simulink model "ModeloSimulink"  (R2023a)
settings: Solver=VariableStepAuto  StartTime=0.0  StopTime=10000  MaxStep=0.1  RelTol=1e-3
settings Model: Creator=User  LastModifiedBy=dougl
settings DebuggingCC: UnconnectedInputMsg=warning  UnconnectedOutputMsg=warning  UnconnectedLineMsg=warning
settings ModelReferenceCC: EnableRefExpFcnMdlSchedulingChecks=on
settings RTWCC: DLArmComputeVersion=19.05

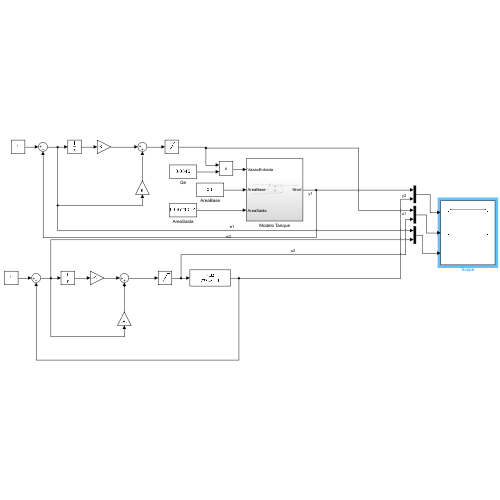
[thumbnail: Simulink's stored preview of the top-level diagram]
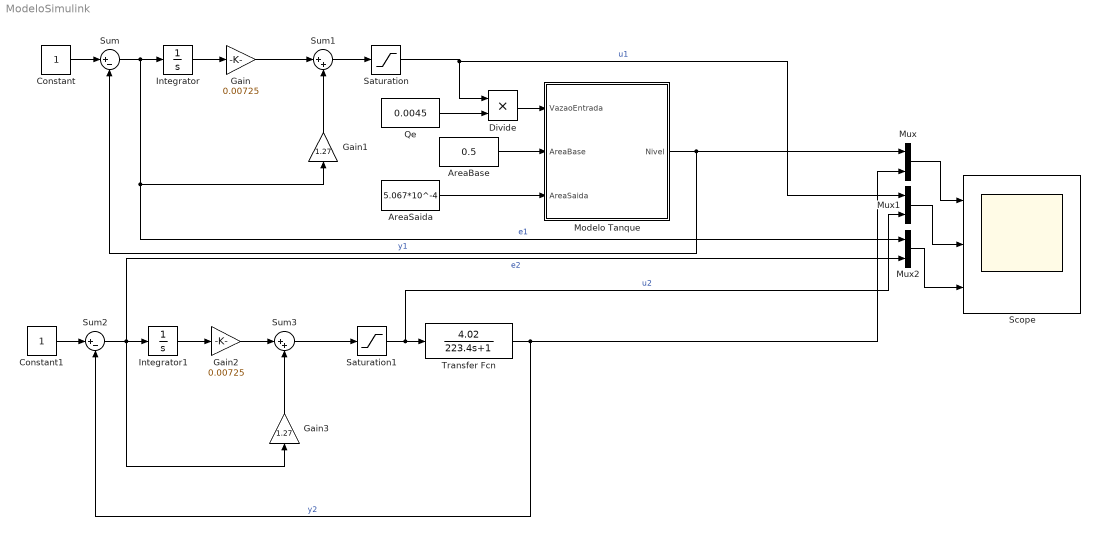
== system ModeloSimulink ==
  AreaBase : Constant  Value=0.5
  AreaSaida : Constant  Value=5.067*10^-4
  Constant : Constant
  Constant1 : Constant
  Divide : Product  Inputs=**
  Gain : Gain  Gain=0.00725
  Gain1 : Gain  Gain=1.27
  Gain2 : Gain  Gain=0.00725
  Gain3 : Gain  Gain=1.27
  Integrator : Integrator
  Integrator1 : Integrator
  Modelo Tanque : Subsystem
  Mux : Mux  Inputs=2
  Mux1 : Mux  Inputs=2
  Mux2 : Mux  Inputs=2
  Qe : Constant  Value=0.0045
  Saturation : Saturate  UpperLimit=1  LowerLimit=0
  Saturation1 : Saturate  UpperLimit=1  LowerLimit=0
  Scope : Scope  NumInputPorts=3
  Sum : Sum  Inputs=|+-
  Sum1 : Sum  Inputs=|++
  Sum2 : Sum  Inputs=|+-
  Sum3 : Sum  Inputs=|++
  Transfer Fcn : TransferFcn  Numerator=[4.02]  Denominator=[223.4 1]
  wires:
  AreaBase/1 -> Modelo Tanque/2(AreaBase)
  AreaSaida/1 -> Modelo Tanque/3(AreaSaida)
  Modelo Tanque/1(Nivel) -> Sum/2, Mux/1  "y1"
  Qe/1 -> Divide/2
  Divide/1 -> Modelo Tanque/1(VazaoEntrada)
  Constant/1 -> Sum/1
  Integrator/1 -> Gain/1
  Gain/1 -> Sum1/1
  Gain1/1 -> Sum1/2
  Saturation/1 -> Mux1/1, Divide/1  "u1"
  Sum/1 -> Mux2/1, Gain1/1, Integrator/1  "e1"
  Sum1/1 -> Saturation/1
  Sum3/1 -> Saturation1/1
  Sum2/1 -> Mux2/2, Integrator1/1, Gain3/1  "e2"
  Gain3/1 -> Sum3/2
  Gain2/1 -> Sum3/1
  Integrator1/1 -> Gain2/1
  Constant1/1 -> Sum2/1
  Transfer Fcn/1 -> Sum2/2, Mux/2  "y2"
  Saturation1/1 -> Mux1/2, Transfer Fcn/1  "u2"
  Mux/1 -> Scope/1
  Mux1/1 -> Scope/2
  Mux2/1 -> Scope/3

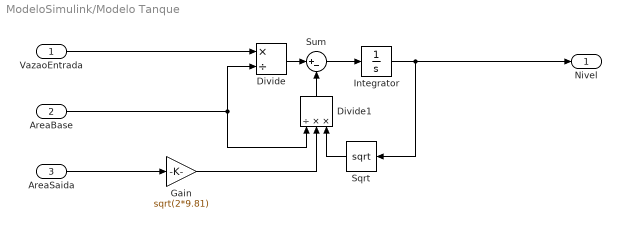
== system ModeloSimulink/Modelo Tanque ==
  VazaoEntrada : Inport
  AreaBase : Inport  Port=2
  AreaSaida : Inport  Port=3
  Divide : Product  Inputs=*/
  Divide1 : Product  Inputs=/**
  Gain : Gain  Gain=sqrt(2*9.81)
  Integrator : Integrator
  Sqrt : Sqrt
  Sum : Sum  Inputs=|+-
  Nivel : Outport
  wires:
  Sqrt/1 -> Divide1/3
  AreaBase/1 -> Divide1/1, Divide/2
  Integrator/1 -> Nivel/1, Sqrt/1
  Sum/1 -> Integrator/1
  VazaoEntrada/1 -> Divide/1
  Divide1/1 -> Sum/2
  Divide/1 -> Sum/1
  AreaSaida/1 -> Gain/1
  Gain/1 -> Divide1/2
